simulink model "Sender"  (R2023b)
settings: Solver=FixedStepAuto  StartTime=0.0  StopTime=20  RelTol=1e-3
libraries: androidsensorlib x2, androidaudiovideolib x1, androidcommunicationlib x1
settings Model: Creator=Swayam  LastModifiedBy=Swayam
settings OptimizationCC: EnhancedBackFolding=on  PassReuseOutputArgsAs=Individual arguments  ZeroExternalMemoryAtStartup=off  ZeroInternalMemoryAtStartup=off  MaxStackSize=64  OptimizeBlockOrder=speed  DifferentSizesBufferReuse=on  OptimizationCustomize=off  EfficientTunableParamExpr=on
settings DebuggingCC: ParameterTunabilityLossMsg=error  IntegerSaturationMsg=none
settings HardwareCC: ProdBitPerLong=64  ProdLargestAtomicInteger=LongLong  ProdLargestAtomicFloat=Double  ProdLongLongMode=on  ProdHWDeviceType=ARM Compatible->ARM 64-bit (LP64)  UseEmbeddedCoderFeatures=off  UseSimulinkCoderFeatures=off
settings SFSimCC: MATLABDynamicMemAlloc=off
settings RTWCC: Description=Embedded Coder  SystemTargetFile=ert.tlc  HardwareBoard=Android Device (64bit)  TLCOptions="-aInlineSetEventsForThisBaseRateFcn=TLC_FALSE -aSuppressMultiTaskScheduler=TLC_FALSE  -aRateBasedStepFcn=0"  TemplateMakefile=ert_default_tmf  RTWVerbose=off  Toolchain=Android SDK/NDK Tools
settings CodeAppCC: ForceParamTrailComments=on  IgnoreCustomStorageClasses=off  OperatorAnnotations=on  SimulinkDataObjDesc=on  SFDataObjDesc=on  InsertBlockDesc=on
settings ERTTargetCC: SupportNonInlinedSFcns=on

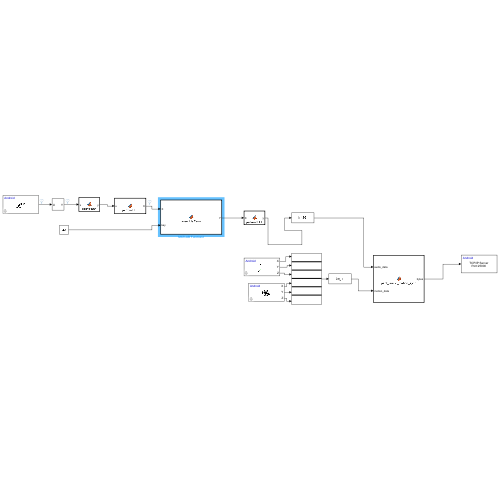
[thumbnail: Simulink's stored preview of the top-level diagram]
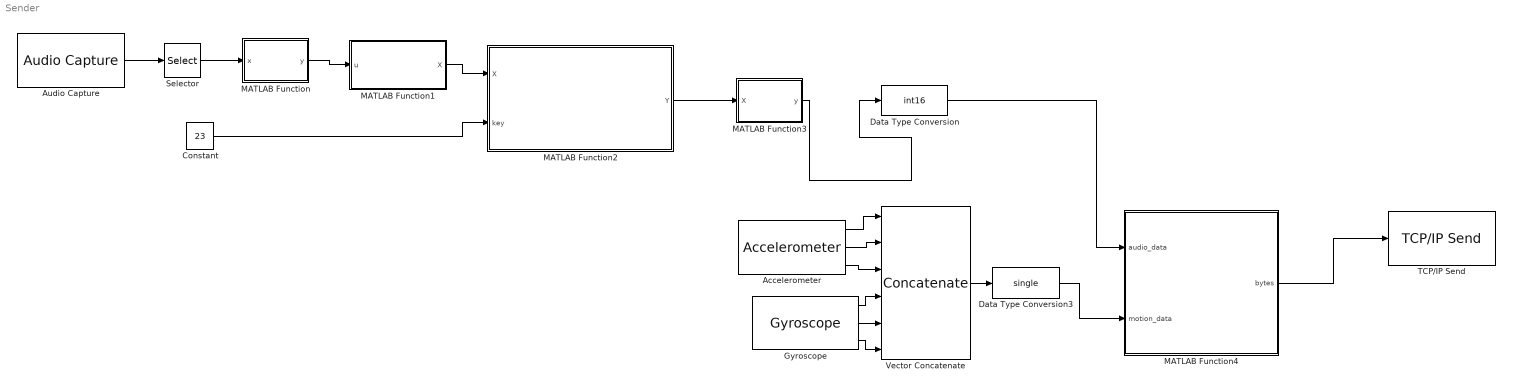
== system Sender ==
  Accelerometer : androidsensorlib/Accelerometer  OutputVector=off  SampleTime=0.1  BlockPlatform=Android
  Audio Capture : androidaudiovideolib/Audio Capture  SampleFreq=44100  FrameSize=4410  SampleTime=0.1  SimulateUsing=Code generation  DeviceStr=0  QueueDuration=0  BlockPlatform=Android  AudioSamplingFreq=44100
  Constant : Constant  Value=23
  Data Type Conversion : DataTypeConversion  OutDataTypeStr=int16  RndMeth=Floor
  Data Type Conversion3 : DataTypeConversion  OutDataTypeStr=single  SaturateOnIntegerOverflow=off  RndMeth=Floor
  Gyroscope : androidsensorlib/Gyroscope  OutputVector=off  SampleTime=0.1  BlockPlatform=Android
  MATLAB Function : MATLAB Function  TreatAsAtomicUnit=on
  MATLAB Function1 : MATLAB Function  TreatAsAtomicUnit=on
  MATLAB Function2 : MATLAB Function  TreatAsAtomicUnit=on
  MATLAB Function3 : MATLAB Function  TreatAsAtomicUnit=on
  MATLAB Function4 : MATLAB Function  TreatAsAtomicUnit=on
  Selector : Selector  NumberOfDimensions=2  InputPortWidth=3  IndexOptions=Select all,Index vector (dialog)  Indices=[1 3],1  OutputSizes=1,1
  TCP/IP Send : androidcommunicationlib/TCP//IP Send  TCPSendId=untitled/TCP//IP_Send  Mode_=Server  LocalServerPort_=25000  RemoteAddr_=127.0.0.1  RemoteServerPort_=25000  ClientPortBindingSelection_=off  ClientPortToBind_=35000  BlockingMode_=off  BlockTimeout_=0.1
  Vector Concatenate : Concatenate  NumInputs=6
  wires:
  MATLAB Function/1(y) -> MATLAB Function1/1(u)
  Audio Capture/1 -> Selector/1
  Selector/1 -> MATLAB Function/1(x)
  MATLAB Function1/1(X) -> MATLAB Function2/1(X)
  MATLAB Function2/1(Y) -> MATLAB Function3/1(X)
  Constant/1 -> MATLAB Function2/2(key)
  MATLAB Function3/1(y) -> Data Type Conversion/1
  Gyroscope/3 -> Vector Concatenate/6
  Gyroscope/2 -> Vector Concatenate/5
  Gyroscope/1 -> Vector Concatenate/4
  Accelerometer/3 -> Vector Concatenate/3
  Accelerometer/2 -> Vector Concatenate/2
  Accelerometer/1 -> Vector Concatenate/1
  Vector Concatenate/1 -> Data Type Conversion3/1
  Data Type Conversion3/1 -> MATLAB Function4/2(motion_data)
  Data Type Conversion/1 -> MATLAB Function4/1(audio_data)
  MATLAB Function4/1(bytes) -> TCP/IP Send/1

== matlab function Sender/MATLAB Function ==
  data: x input; y output
function y = applyHann(x)

x = double(x);
[N,C] = size(x);
n = (0:N-1)';                        % column
w = 0.5 - 0.5*cos(2*pi*n/(N-1));     % Hann
y = x .* repmat(w,1,C);              % element-wise multiply
end

== matlab function Sender/MATLAB Function1 ==
  data: u input; X output
function X = performFFT(u)


x = complex(double(u));          % avoid complex–integer issues
N = size(x,1);                   % FFT length = frame length
X = fft(x, N, 1);                % FFT along dim-1 (rows)
end

== matlab function Sender/MATLAB Function2 ==
  data: X input; Y output; key input
function Y = scramblePerm(X, key)

[N,C] = size(X);
Y = complex(zeros(N,C,'like',X));


posIdx = 2:N/2;                
negIdx = N - posIdx + 2;       
K = numel(posIdx);  if K==0, Y = X; return; end


state = hash_key(uint8(key));
state = bitxor(state, uint32(N));


perm = scrambling(state, K);
pidx = posIdx(perm);

Y(posIdx,:)      = X(pidx,:);
Y(negIdx,:)      = conj(Y(posIdx,:));
Y([1, N/2+1], :) = X([1, N/2+1], :);   % keep DC & Nyquist
end

function seed = hash_key(keyBytes)
b0=uint32(0); b1=uint32(0); b2=uint32(0); b3=uint32(0);
if numel(keyBytes)>=1, b0 = uint32(keyBytes(1)); end
if numel(keyBytes)>=2, b1 = bitshift(uint32(keyBytes(2)),  8); end
if numel(keyBytes)>=3, b2 = bitshift(uint32(keyBytes(3)), 16); end
if numel(keyBytes)>=4, b3 = bitshift(uint32(keyBytes(4)), 24); end
seed = bitor(bitor(b0,b1), bitor(b2,b3));
if seed==0, seed = uint32(1); end
end

function perm = scrambling(state, K)
% Fisher–Yates using multiply-high to avoid modulo bias
perm = 1:K;
for i = K:-1:2
    [state, r] = xorshift32(state);
    j = double(bitshift(uint64(r)*uint64(i), -32)) + 1;  % 1..i
    t = perm(i);
    perm(i) = perm(j); 
    perm(j) = t;
end
end

function [state, r] = xorshift32(state)
state = bitxor(state, bitshift(state, 13));
state = bitxor(state, bitshift(state, -17));
state = bitxor(state, bitshift(state, 5));
r = state;  % uint32
end

== matlab function Sender/MATLAB Function3 ==
  data: X input; y output
function y = performIFFT(X)

Xc = complex(double(X));          % ensure complex double
N  = size(Xc,1);
y  = real(ifft(Xc, N, 1));        % IFFT along rows (frame length)
end

== matlab function Sender/MATLAB Function4 ==
  data: audio_data input; bytes output; motion_data input
function bytes = pack_audio_motion_sync(audio_data, motion_data)
%#codegen
assert(numel(audio_data)==4410 && isa(audio_data,'int16'));
assert(numel(motion_data)==6      && isa(motion_data,'single'));
assert(isscalar(t_ms)         && isa(t_ms,'uint32'));
bytes = zeros(8848,1,'uint8');
bytes(5:28)     = typecast(single(motion_data(:)).', 'uint8');   % 24
bytes(29:8848)  = typecast(audio_data(:), 'uint8');           % 8820
end
